simulink model "testingPLUT"  (R2019b)
settings: Solver=VariableStepAuto  StartTime=0.0  StopTime=stop_time  RelTol=1e-3
values from neighbouring files (symbols this model uses):
  X_in = zeros(1, 2^(M_bits+N_bits))    [PLUTtest2_reprogramming.m]    (also in TestingLibraryScripts.m = X_LUT; testingTEMP.m)
libraries: DSP_FPGA_Accelerated_Toolbox x1
settings Model: Creator=Bailey  LastModifiedBy=Balad
settings SFSimCC: CustomCodeUndefinedFunction=UseInterfaceOnly

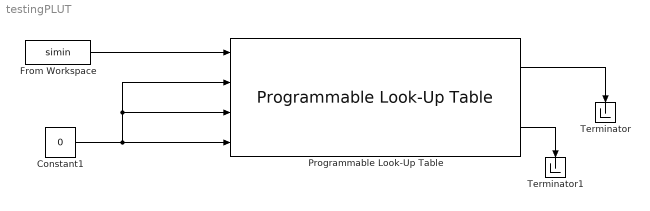
== system testingPLUT ==
  Constant1 : Constant  Value=0  SampleTime=1/48000
  From Workspace : FromWorkspace  VariableName=simin  SampleTime=0
  Programmable Look-Up Table : DSP_FPGA_Accelerated_Toolbox/Programmable Look-Up Table  TableFn=X_in.^0.5  maxInput=2  floor_in_tab=2^-15  error_cap_tab=0.02  ERR_DIAG=on  N_bits_tab=4  M_bits_tab=5  igotthis=off  Table_Init=0  d=0
      settings: SourceProductName=DSP FPGA Accelerated Toolbox
  Terminator : Terminator
  Terminator1 : Terminator
  wires:
  Programmable Look-Up Table/1 -> Terminator/1
  Programmable Look-Up Table/2 -> Terminator1/1
  Constant1/1 -> Programmable Look-Up Table/3, Programmable Look-Up Table/2, Programmable Look-Up Table/4
  From Workspace/1 -> Programmable Look-Up Table/1
